simulink model "Three_Phase_Inverter_Model"  (R2020a)
settings: Solver=VariableStepAuto  StartTime=0.0  StopTime=5/60  RelTol=1e-3
libraries: powerlib x12
settings Model: Creator=Ricardo Romero  LastModifiedBy=Ricardo Romero

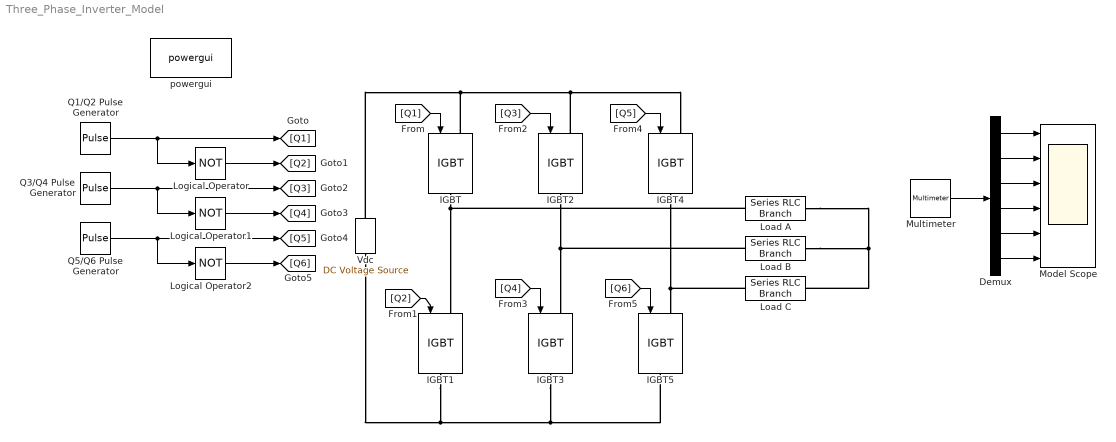
== system Three_Phase_Inverter_Model ==
  Demux : Demux  Outputs=6
  IGBT{,1..5} (6 alike) : powerlib/Power Electronics/IGBT  Ron=0.001  Lon=0  Vf=1  Tf=1e-6  Tt=2e-6  IC=0  Rs=1e5  Cs=inf  Measurements=off
  Load A : powerlib/Elements/Series RLC Branch  LConnTagsString=__new0  RConnTagsString=__new0  BranchType=R  Resistance=10  Inductance=1e-3  SetiL0=off  InitialCurrent=0  Capacitance=1e-6  Setx0=off  InitialVoltage=0  Measurements=Branch voltage and current
  Load B : powerlib/Elements/Series RLC Branch  LConnTagsString=__new0  RConnTagsString=__new0  BranchType=R  Resistance=10  Inductance=1e-3  SetiL0=off  InitialCurrent=0  Capacitance=1e-6  Setx0=off  InitialVoltage=0  Measurements=Branch voltage and current
  Load C : powerlib/Elements/Series RLC Branch  LConnTagsString=__new0  RConnTagsString=__new0  BranchType=R  Resistance=10  Inductance=1e-3  SetiL0=off  InitialCurrent=0  Capacitance=1e-6  Setx0=off  InitialVoltage=0  Measurements=Branch voltage and current
  Logical Operator : Logic  Operator=NOT  AllPortsSameDT=off  OutDataTypeStr=boolean
  Logical Operator1 : Logic  Operator=NOT  AllPortsSameDT=off  OutDataTypeStr=boolean
  Logical Operator2 : Logic  Operator=NOT  AllPortsSameDT=off  OutDataTypeStr=boolean
  Model Scope : Scope  NumInputPorts=6
  Multimeter : powerlib/Measurements/Multimeter  PhasorSimulation=off  OutputType=Complex  sel=[2 3 1 5 6 4]  L=6  Gain=[1 1 1 1 1 1]  yselected={'Ub: Load A','Ub: Load B','Ub: Load C','Ib: Load A','Ib: Load B','Ib: Load C'};  PSBOutputType=1  PSBequivalent=0  AxesSetting=[0,0.1,-100,100]  Display=0  SavedBlockNames=-11
  Q1/Q2 Pulse Generator : DiscretePulseGenerator  PulseType=Time based  Period=1/60  PulseWidth=50
  Q3/Q4 Pulse Generator : DiscretePulseGenerator  PulseType=Time based  Period=1/60  PulseWidth=50  PhaseDelay=-240/360*(1/60)
  Q5/Q6 Pulse Generator : DiscretePulseGenerator  PulseType=Time based  Period=1/60  PulseWidth=50  PhaseDelay=-(120/360)*(1/60)
  Vdc : powerlib/Electrical Sources/DC Voltage Source  Amplitude=100  Measurements=None
  powergui : powerlib/powergui  Priority=1  SimulationMode=Continuous  SampleTime=50e-6  frequency=60  Iterations=50  frequencyindice=0  Pbase=100e6  ErrMax=1e-4  UnitsV=kV  UnitsW=MW  buscounter=0  FunctionMessages=off  echomessages=off  EnableUseOfTLC=off  CurrentSourceSwitches=off  DisableSnubberDevices=off  DisableRonSwitches=off  DisableVfSwitches=off  DisplayEquations=off  AutomaticDiscreteSolvers=off  SolverType=Tustin/Backward Euler (TBE)  Interpol=off  ExternalGateDelay=off  methode=off  Ts=100  x0status=blocks  SPID=on  SwTol=0  HookPort=off  NonlinearTolerance=1e-4  nMaxIteration=100  ContinueOnMaxIteration=off  RestoreLinks=warning  ResistiveCurrentMeasurement=off  Frange=[0:2:500]  Ylog=off  Xlog=on  ShowGrid=off  save=off  variable=ZData  structure=0  ZoomFFT=off  StartTime=0.0  cycles=1  DisplayStyle=1  fundamental=60  FreqAxis=off  MaxFrequency=1000  frequencyindicesteady=1  RmsSteady=1  display=off
  wires:
  Q5/Q6 Pulse Generator/1 -> [Q5], Logical Operator2/1
  Q3/Q4 Pulse Generator/1 -> Logical Operator1/1, [Q3]
  Q1/Q2 Pulse Generator/1 -> [Q1], Logical Operator/1
  Logical Operator/1 -> [Q2]
  Logical Operator1/1 -> [Q4]
  Logical Operator2/1 -> [Q6]
  [Q1] -> IGBT/1
  [Q2] -> IGBT1/1
  [Q3] -> IGBT2/1
  [Q4] -> IGBT3/1
  [Q5] -> IGBT4/1
  [Q6] -> IGBT5/1
  Multimeter/1 -> Demux/1
  Demux/1 -> Model Scope/1
  Demux/2 -> Model Scope/2
  Demux/3 -> Model Scope/3
  Demux/4 -> Model Scope/4
  Demux/5 -> Model Scope/5
  Demux/6 -> Model Scope/6
  connections:
  IGBT/RConn1 -- IGBT1/LConn1 -- Load A/LConn1
  IGBT2/RConn1 -- Load B/LConn1 -- IGBT3/LConn1
  IGBT4/RConn1 -- Load C/LConn1 -- IGBT5/LConn1
  Vdc/RConn1 -- IGBT/LConn1 -- IGBT2/LConn1 -- IGBT4/LConn1
  Vdc/LConn1 -- IGBT1/RConn1 -- IGBT3/RConn1 -- IGBT5/RConn1
  Load A/RConn1 -- Load B/RConn1 -- Load C/RConn1
